simulink model "PMSM_FOC_Baseline"  (R2025b)
settings: Solver=FixedStepDiscrete  StartTime=0.0  StopTime=4  FixedStep=0.0001  RelTol=1e-3
settings Model: Creator=Wu  LastModifiedBy=Wu
settings DataIOCC: SaveFormat=StructureWithTime  SignalLogging=off

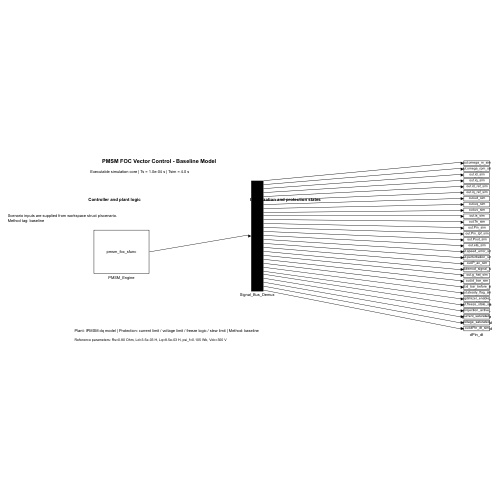
[thumbnail: Simulink's stored preview of the top-level diagram]
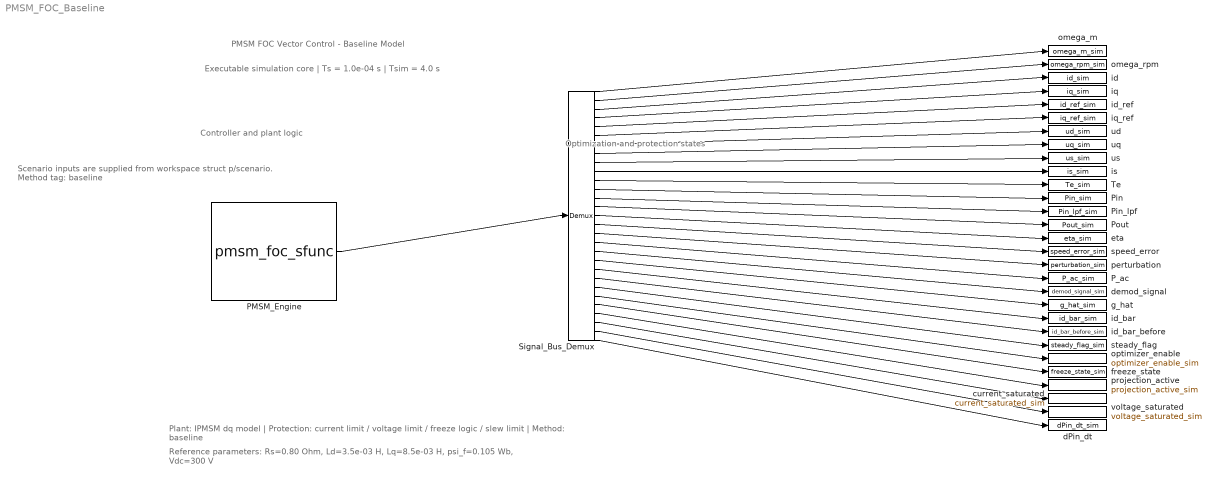
== system PMSM_FOC_Baseline ==
  note: PMSM FOC Vector Control - Baseline Model
  note: Executable simulation core | Ts = 1.0e-04 s | Tsim = 4.0 s
  note: Controller and plant logic
  note: Optimization and protection states
  note: Plant: IPMSM dq model | Protection: current limit / voltage limit / freeze logic / slew limit | Method: baseline
  note: Reference parameters: Rs=0.80 Ohm, Ld=3.5e-03 H, Lq=8.5e-03 H, psi_f=0.105 Wb, Vdc=300 V
  note: Scenario inputs are supplied from workspace struct p/scenario.
      | Method tag: baseline
  PMSM_Engine : M-S-Function  FunctionName=pmsm_foc_sfunc  Parameters=p, 'baseline', scenario
  P_ac : ToWorkspace  VariableName=P_ac_sim  SaveFormat=Timeseries  SampleTime=-1
  Pin : ToWorkspace  VariableName=Pin_sim  SaveFormat=Timeseries  SampleTime=-1
  Pin_lpf : ToWorkspace  VariableName=Pin_lpf_sim  SaveFormat=Timeseries  SampleTime=-1
  Pout : ToWorkspace  VariableName=Pout_sim  SaveFormat=Timeseries  SampleTime=-1
  Signal_Bus_Demux : Demux  Outputs=29
  Te : ToWorkspace  VariableName=Te_sim  SaveFormat=Timeseries  SampleTime=-1
  current_saturated : ToWorkspace  VariableName=current_saturated_sim  SaveFormat=Timeseries  SampleTime=-1
  dPin_dt : ToWorkspace  VariableName=dPin_dt_sim  SaveFormat=Timeseries  SampleTime=-1
  demod_signal : ToWorkspace  VariableName=demod_signal_sim  SaveFormat=Timeseries  SampleTime=-1
  eta : ToWorkspace  VariableName=eta_sim  SaveFormat=Timeseries  SampleTime=-1
  freeze_state : ToWorkspace  VariableName=freeze_state_sim  SaveFormat=Timeseries  SampleTime=-1
  g_hat : ToWorkspace  VariableName=g_hat_sim  SaveFormat=Timeseries  SampleTime=-1
  id : ToWorkspace  VariableName=id_sim  SaveFormat=Timeseries  SampleTime=-1
  id_bar : ToWorkspace  VariableName=id_bar_sim  SaveFormat=Timeseries  SampleTime=-1
  id_bar_before : ToWorkspace  VariableName=id_bar_before_sim  SaveFormat=Timeseries  SampleTime=-1
  id_ref : ToWorkspace  VariableName=id_ref_sim  SaveFormat=Timeseries  SampleTime=-1
  iq : ToWorkspace  VariableName=iq_sim  SaveFormat=Timeseries  SampleTime=-1
  iq_ref : ToWorkspace  VariableName=iq_ref_sim  SaveFormat=Timeseries  SampleTime=-1
  is : ToWorkspace  VariableName=is_sim  SaveFormat=Timeseries  SampleTime=-1
  omega_m : ToWorkspace  VariableName=omega_m_sim  SaveFormat=Timeseries  SampleTime=-1
  omega_rpm : ToWorkspace  VariableName=omega_rpm_sim  SaveFormat=Timeseries  SampleTime=-1
  optimizer_enable : ToWorkspace  VariableName=optimizer_enable_sim  SaveFormat=Timeseries  SampleTime=-1
  perturbation : ToWorkspace  VariableName=perturbation_sim  SaveFormat=Timeseries  SampleTime=-1
  projection_active : ToWorkspace  VariableName=projection_active_sim  SaveFormat=Timeseries  SampleTime=-1
  speed_error : ToWorkspace  VariableName=speed_error_sim  SaveFormat=Timeseries  SampleTime=-1
  steady_flag : ToWorkspace  VariableName=steady_flag_sim  SaveFormat=Timeseries  SampleTime=-1
  ud : ToWorkspace  VariableName=ud_sim  SaveFormat=Timeseries  SampleTime=-1
  uq : ToWorkspace  VariableName=uq_sim  SaveFormat=Timeseries  SampleTime=-1
  us : ToWorkspace  VariableName=us_sim  SaveFormat=Timeseries  SampleTime=-1
  voltage_saturated : ToWorkspace  VariableName=voltage_saturated_sim  SaveFormat=Timeseries  SampleTime=-1
  wires:
  PMSM_Engine/1 -> Signal_Bus_Demux/1
  Signal_Bus_Demux/1 -> omega_m/1
  Signal_Bus_Demux/2 -> omega_rpm/1
  Signal_Bus_Demux/3 -> id/1
  Signal_Bus_Demux/4 -> iq/1
  Signal_Bus_Demux/5 -> id_ref/1
  Signal_Bus_Demux/6 -> iq_ref/1
  Signal_Bus_Demux/7 -> ud/1
  Signal_Bus_Demux/8 -> uq/1
  Signal_Bus_Demux/9 -> us/1
  Signal_Bus_Demux/10 -> is/1
  Signal_Bus_Demux/11 -> Te/1
  Signal_Bus_Demux/12 -> Pin/1
  Signal_Bus_Demux/13 -> Pin_lpf/1
  Signal_Bus_Demux/14 -> Pout/1
  Signal_Bus_Demux/15 -> eta/1
  Signal_Bus_Demux/16 -> speed_error/1
  Signal_Bus_Demux/17 -> perturbation/1
  Signal_Bus_Demux/18 -> P_ac/1
  Signal_Bus_Demux/19 -> demod_signal/1
  Signal_Bus_Demux/20 -> g_hat/1
  Signal_Bus_Demux/21 -> id_bar/1
  Signal_Bus_Demux/22 -> id_bar_before/1
  Signal_Bus_Demux/23 -> steady_flag/1
  Signal_Bus_Demux/24 -> optimizer_enable/1
  Signal_Bus_Demux/25 -> freeze_state/1
  Signal_Bus_Demux/26 -> projection_active/1
  Signal_Bus_Demux/27 -> current_saturated/1
  Signal_Bus_Demux/28 -> voltage_saturated/1
  Signal_Bus_Demux/29 -> dPin_dt/1
